simulink model "task_3"  (R2023a)
settings: Solver=VariableStepAuto  StartTime=0.0  StopTime=50  RelTol=1e-8
settings Model: Creator=user  LastModifiedBy=user

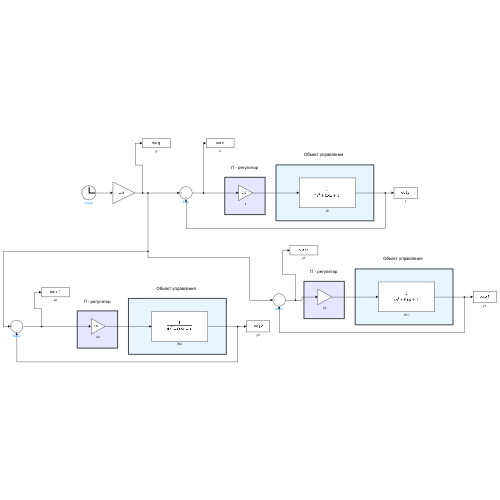
[thumbnail: Simulink's stored preview of the top-level diagram]
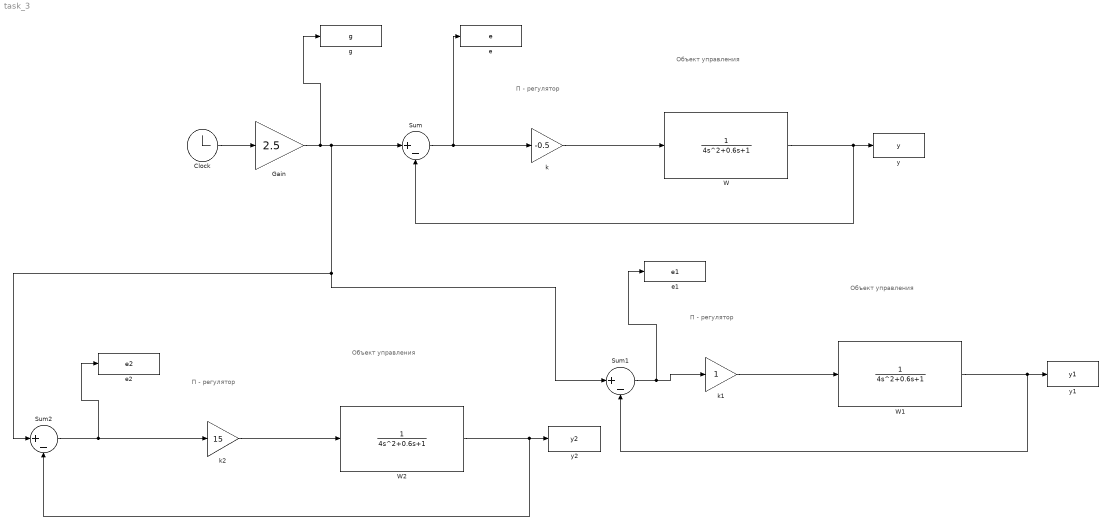
== system task_3 ==
  note: Объект управления
  note: П - регулятор
  note: П - регулятор
  note: Объект управления
  note: П - регулятор
  note: Объект управления
  Clock : Clock
  Gain : Gain  Gain=2.5
  Sum : Sum  Inputs=|+-
  Sum1 : Sum  Inputs=|+-
  Sum2 : Sum  Inputs=|+-
  W : TransferFcn  Denominator=[4 0.6 1]
  W1 : TransferFcn  Denominator=[4 0.6 1]
  W2 : TransferFcn  Denominator=[4 0.6 1]
  e : ToWorkspace  VariableName=e  SaveFormat=Timeseries  SampleTime=-1
  e1 : ToWorkspace  VariableName=e1  SaveFormat=Timeseries  SampleTime=-1
  e2 : ToWorkspace  VariableName=e2  SaveFormat=Timeseries  SampleTime=-1
  g : ToWorkspace  VariableName=g  SaveFormat=Timeseries  SampleTime=-1
  k : Gain  Gain=-0.5
  k1 : Gain
  k2 : Gain  Gain=15
  y : ToWorkspace  VariableName=y  SaveFormat=Timeseries  SampleTime=-1
  y1 : ToWorkspace  VariableName=y1  SaveFormat=Timeseries  SampleTime=-1
  y2 : ToWorkspace  VariableName=y2  SaveFormat=Timeseries  SampleTime=-1
  wires:
  Sum/1 -> e/1, k/1
  k/1 -> W/1
  W/1 -> Sum/2, y/1
  Gain/1 -> g/1, Sum1/1, Sum2/1, Sum/1
  W1/1 -> Sum1/2, y1/1
  Sum1/1 -> e1/1, k1/1
  k1/1 -> W1/1
  W2/1 -> Sum2/2, y2/1
  Sum2/1 -> e2/1, k2/1
  k2/1 -> W2/1
  Clock/1 -> Gain/1
